simulink model "APLRL2D_avoidance_version"  (R2020a)
settings: Solver=ode23t  StartTime=0.0  StopTime=Tf  RelTol=1e-2  EnableMultiTasking=on
PreLoadFcn:
  | robotParametersRL
undefined symbols (not defined in the file or in its folder): Angular, Linear, Pose
libraries: robotlib x12, simulink x6, sharedtransform x1, rllib x1
(part 1 of 2)
settings Model: EnablePacing=on  Creator=scastro  LastModifiedBy=apl
settings SolverCC: ZeroCrossAlgorithm=Adaptive
settings DataIOCC: SaveOutput=off  SignalLogging=off  DSMLogging=off  SaveTime=off  ReturnWorkspaceOutputs=off  OutputTimes=0:0.01:10
settings OptimizationCC: LifeSpan=inf
settings DebuggingCC: MaxConsecutiveZCsMsg=warning  IgnoredZcDiagnostic=none  ParameterPrecisionLossMsg=none  AllowSymbolicDim=off  SFUnexpectedBacktrackingDiag=warning  SFNoUnconditionalDefaultTransitionDiag=warning  SFExecutionAtInitializationDiag=none  UnitsInconsistencyMsg=none  ArithmeticOperatorsInVariantConditions=warning
settings SFSimCC: SimUseLocalCustomCode=off  CustomCodeUndefinedFunction=UseInterfaceOnly
settings RTWCC: RTWUseLocalCustomCode=off
settings CodeAppCC: StateflowObjectComments=on
settings GRTTargetCC: TargetLangStandard=C89/C90 (ANSI)
settings ConfigComp: CovMetricSettings=dw  CovHtmlReporting=on  CovSaveCumulativeToWorkspaceVar=on  CovSaveSingleToWorkspaceVar=on  CovExternalEMLEnable=off  CovSFcnEnable=off
settings SimscapeCC: SimscapeNormalizeSystem=off  SimscapeLogOpenViewer=on  SimscapeLogLimitData=off  SimscapeLogDataHistory=10000
settings ConfigurationSet: Description=SimMechanics 2G
settings DiagnosticsConfigSet: SimMechanicsRigidlyBoundBlock=none
settings ExplorerConfigSet: InternalSimMechanicsExplorerSettings="<ExplorerConfiguration><canonicalview>default</canonicalview><AnimationSetting><BasePlaybackSpeed>1.0</BasePlaybackSpeed><PlaybackSpeedFactor>1.0</PlaybackSpeedFactor></AnimationSetting><TilePanel><TileInfo><Tiles Columns=\"1\" Count=\"1\" Rows=\"1\"><Column Weight=\"1\"/><Row Weight=\"1\"/><Tile Height=\"1\" Width=\"1\" X=\"0\" Y=\"0\"/></Tiles></TileInfo><SceneInfo><SceneViewer><BGColor><R>0.60000002384185791</R><G>0.60000002384185791</G><B>0.60000002384185791</B></BGColor><Camera><DoPerspective>off</DoPerspective><Position><X>8.91370771296205788</X><Y>-7.80792633437846995</Y><Z>7.38233363180041291</Z></Position><Center><X>2.84109241733315354</X><Y>0.225363634109725985</Y><Z>-0.303011043015117276</Z></Center><Up><X>-0.335329266167064488</X><Y>0.506481739462631531</Y><Z>0.79437430147428989</Z></Up><ViewLimDist>1</ViewLimDist><YLim>1.70039015453236564</YLim><XLim>2.75119305901865907</XLim></Camera></SceneViewer></SceneInfo></TilePanel><MechEditorPanel><Cameras/><GfxPanelCameraMap/><VideoCreator><PlaybackSpeedRatio>1.0</PlaybackSpeedRatio><FrameRate>30</FrameRate><VideoFormat>Motion JPEG AVI</VideoFormat><FrameSize>auto</FrameSize></VideoCreator></MechEditorPanel></ExplorerConfiguration>"

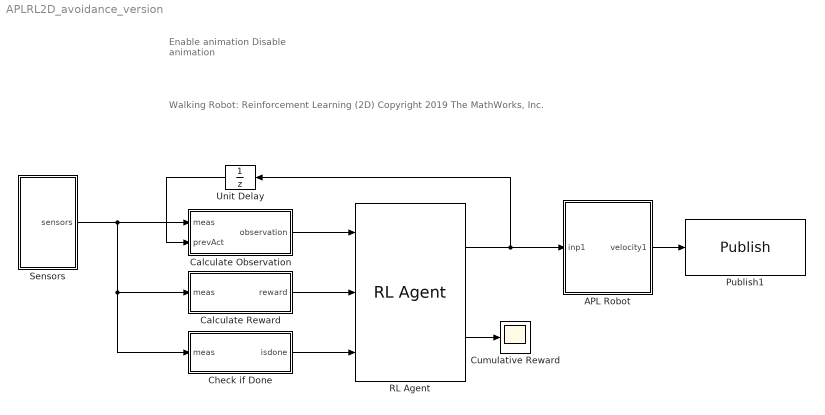
== system APLRL2D_avoidance_version ==
  note: Enable animation
      |
      | Disable animation
  note: Walking Robot: Reinforcement Learning (2D)
      |
      | Copyright 2019 The MathWorks, Inc.
  APL Robot : Subsystem
  Calculate Observation : Subsystem
  Calculate Reward : Subsystem
  Check if Done : Subsystem
  Cumulative Reward : Scope
  Publish1 : robotlib/Publish  topicSource=Select from ROS network  topic=/cmd_vel  messageType=geometry_msgs/Twist  messageQueueLength=10
  RL Agent : rllib/RL Agent  Agent=agent  ProvideReward=on  ProvideIsDone=on  ProvideCumRwd=on  TreatAsDirectFeedthrough=on  CollectLoggedSignals=on  CollectModelStates=on
      settings: SourceProductName=Reinforcement Learning
  Sensors : Subsystem
  Unit Delay : UnitDelay  SampleTime=-1  HasFrameUpgradeWarning=on
  wires:
  Calculate Reward/1(reward) -> RL Agent/2
  Calculate Observation/1(observation) -> RL Agent/1
  Check if Done/1(isdone) -> RL Agent/3
  RL Agent/2 -> Cumulative Reward/1
  Unit Delay/1 -> Calculate Observation/2(prevAct)
  APL Robot/1(velocity1) -> Publish1/1
  RL Agent/1 -> Unit Delay/1, APL Robot/1(inp1)
  Sensors/1(sensors) -> Check if Done/1(meas), Calculate Reward/1(meas), Calculate Observation/1(meas)

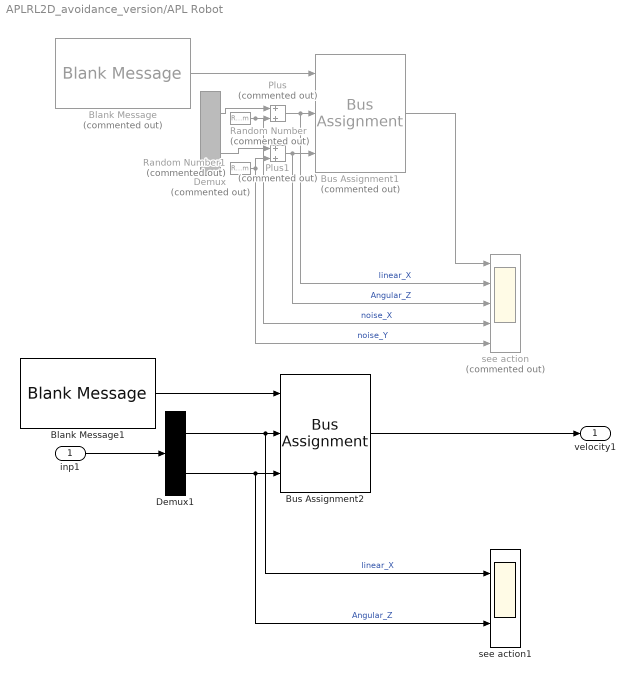
== system APLRL2D_avoidance_version/APL Robot ==
  inp1 : Inport
  Blank Message : robotlib/Blank Message  Commented=on  messageClass=Message  entityType=geometry_msgs/Twist  messageType=geometry_msgs/Twist  SampleTime=inf
  Blank Message1 : robotlib/Blank Message  messageClass=Message  entityType=geometry_msgs/Twist  messageType=geometry_msgs/Twist  SampleTime=inf
  Bus Assignment1 : BusAssignment  Commented=on  AssignedSignals=Linear.X,Angular.Z
  Bus Assignment2 : BusAssignment  AssignedSignals=Linear.X,Angular.Z
  Demux : Demux  Commented=on  Outputs=2
  Demux1 : Demux  Outputs=2
  Plus : Sum  Commented=on
  Plus1 : Sum  Commented=on
  Random Number : RandomNumber  Commented=on  Variance=0.005625  Seed=1  SampleTime=0.1
  Random Number1 : RandomNumber  Commented=on  Variance=0.005625  SampleTime=0.1
  see action : Scope  Commented=on  NumInputPorts=5
  see action1 : Scope  NumInputPorts=2
  velocity1 : Outport  VectorParamsAs1DForOutWhenUnconnected=off
  wires:
  Demux/2 -> Plus1/1
  Demux/1 -> Plus/1
  Blank Message/1 -> Bus Assignment1/1
  Bus Assignment1/1 -> see action/1
  Plus/1 -> see action/2, Bus Assignment1/2  "linear_X"
  Random Number/1 -> see action/4, Plus/2  "noise_X"
  Random Number1/1 -> see action/5, Plus1/2  "noise_Y"
  Plus1/1 -> see action/3, Bus Assignment1/3  "Angular_Z"
  Demux1/1 -> see action1/1, Bus Assignment2/2  "linear_X"
  Demux1/2 -> see action1/2, Bus Assignment2/3  "Angular_Z"
  Blank Message1/1 -> Bus Assignment2/1
  Bus Assignment2/1 -> velocity1/1
  inp1/1 -> Demux1/1

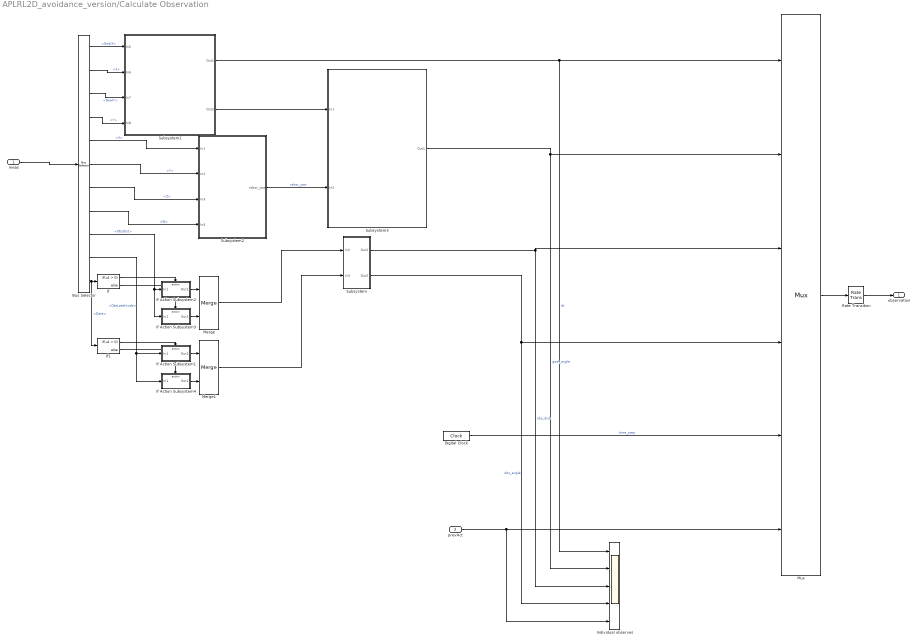
== system APLRL2D_avoidance_version/Calculate Observation ==
  meas : Inport
  prevAct : Inport  Port=2
  Bus Selector : BusSelector  OutputSignals=signal2.GoalX,signal3.Pose.Pose.Position.X,signal2.GoalY,signal3.Pose.Pose.Position.Y,signal3.Pose.Pose.Orientation.X,signal3.Pose.Pose.Orientation.Y,signal3.Pose.Pose.Orientation.Z,signal3.Pose.Pose.Orientation.W,signal2.ObsDist,signal2.ObsLatelitude,signal1.Data
  Digital Clock : DigitalClock  SampleTime=0.1
  If : If
  If Action Subsystem1 : Subsystem  TreatAsAtomicUnit=on
  If Action Subsystem2 : Subsystem  TreatAsAtomicUnit=on
  If Action Subsystem3 : Subsystem  TreatAsAtomicUnit=on
  If Action Subsystem4 : Subsystem  TreatAsAtomicUnit=on
  If1 : If
  Individual observes : Scope  NumInputPorts=5
  Merge : Merge
  Merge1 : Merge
  Mux : Mux  Inputs=6
  Rate Transition : RateTransition
  Subsystem : Subsystem
  Subsystem1 : Subsystem
  Subsystem2 : Subsystem
  Subsystem3 : Subsystem
  observation : Outport  VectorParamsAs1DForOutWhenUnconnected=off
  wires:
  meas/1 -> Bus Selector/1
  Mux/1 -> Rate Transition/1
  prevAct/1 -> Individual observes/5, Mux/6
  Rate Transition/1 -> observation/1
  Digital Clock/1 -> Mux/5  "time_step"
  Bus Selector/2 -> Subsystem1/2(In6)  "<X>"
  Bus Selector/4 -> Subsystem1/4(In8)  "<Y>"
  Bus Selector/1 -> Subsystem1/1(In5)  "<GoalX>"
  Bus Selector/3 -> Subsystem1/3(In7)  "<GoalY>"
  Subsystem1/1(Out1) -> Individual observes/1, Mux/1  "dt"
  Bus Selector/8 -> Subsystem2/4(In4)  "<W>"
  Bus Selector/7 -> Subsystem2/3(In3)  "<Z>"
  Bus Selector/6 -> Subsystem2/2(In2)  "<Y>"
  Bus Selector/5 -> Subsystem2/1(In1)  "<X>"
  Subsystem1/2(Out2) -> Subsystem3/1(In1)
  Subsystem3/1(Out1) -> Individual observes/2, Mux/2  "goal_angle"
  Bus Selector/9 -> If Action Subsystem3/1(In1), If Action Subsystem2/1(In1)  "<ObsDist>"
  Subsystem/1(Out1) -> Individual observes/3, Mux/3  "obs_dist"
  Subsystem/2(Out2) -> Individual observes/4, Mux/4  "obs_angle"
  Subsystem2/1(robot_yaw) -> Subsystem3/2(In2)  "robot_yaw"
  Merge/1 -> Subsystem/1(In2)
  Merge1/1 -> Subsystem/2(In3)
  Bus Selector/11 -> If1/1, If/1  "<Data>"
  If/1 -> If Action Subsystem2/Action
  If/2 -> If Action Subsystem3/Action
  If Action Subsystem2/1(Out1) -> Merge/1
  If Action Subsystem3/1(Out1) -> Merge/2
  If Action Subsystem1/1(Out1) -> Merge1/1
  If1/2 -> If Action Subsystem4/Action
  If Action Subsystem4/1(Out1) -> Merge1/2
  If1/1 -> If Action Subsystem1/Action
  Bus Selector/10 -> If Action Subsystem1/1(In1), If Action Subsystem4/1(In1)  "<ObsLatelitude>"

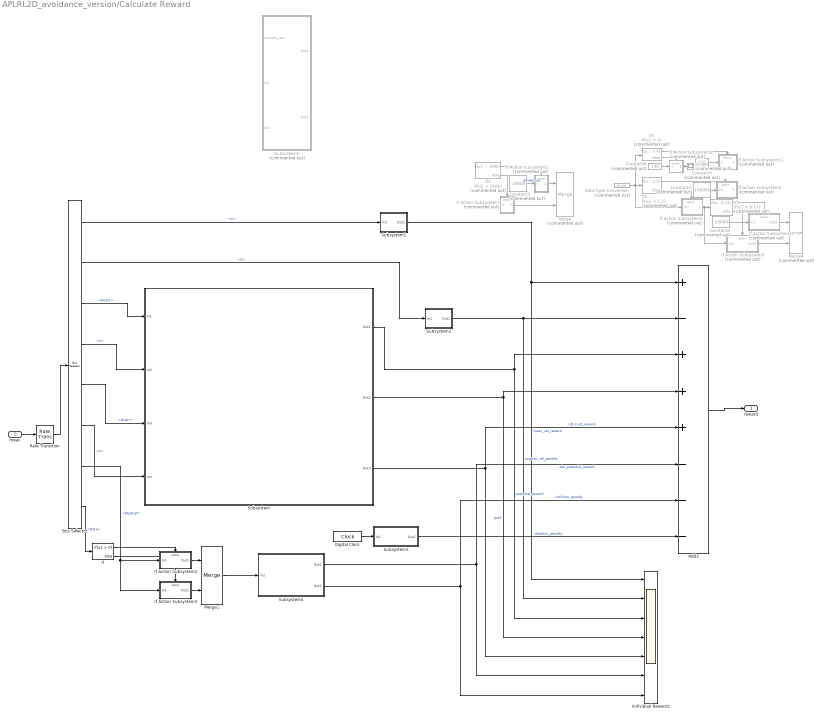
== system APLRL2D_avoidance_version/Calculate Reward ==
  meas : Inport
  Add2 : Sum  Inputs=+-+++---
  Bus Selector : BusSelector  OutputSignals=signal3.Twist.Twist.Linear.X,signal3.Twist.Twist.Angular.Z,signal2.GoalX,signal3.Pose.Pose.Position.X,signal2.GoalY,signal3.Pose.Pose.Position.Y,signal2.ObsDist,signal1.Data
  Constant2 : Constant  Commented=on  Value=100000
  Constant3 : Constant  Commented=on  Value=-10000
  Constant4 : Constant  Commented=on  Value=10000
  Constant5 : Constant  Commented=on  Value=100
  Constant6 : Constant  Commented=on  Value=100
  Data Type Conversion : DataTypeConversion  Commented=on  OutDataTypeStr=double
  Digital Clock : DigitalClock  SampleTime=0.1
  If : If
  If Action Subsystem1 : Subsystem  Commented=on  TreatAsAtomicUnit=on
  If Action Subsystem10 : Subsystem  Commented=on  TreatAsAtomicUnit=on
  If Action Subsystem11 : Subsystem  Commented=on  TreatAsAtomicUnit=on
  If Action Subsystem2 : Subsystem  TreatAsAtomicUnit=on
  If Action Subsystem3 : Subsystem  TreatAsAtomicUnit=on
  If Action Subsystem5 : Subsystem  Commented=on  TreatAsAtomicUnit=on
  If Action Subsystem6 : Subsystem  Commented=on  TreatAsAtomicUnit=on
  If Action Subsystem7 : Subsystem  Commented=on  TreatAsAtomicUnit=on
  If Action Subsystem8 : Subsystem  Commented=on  TreatAsAtomicUnit=on
  If Action Subsystem9 : Subsystem  Commented=on  TreatAsAtomicUnit=on
  If2 : If  Commented=on  IfExpression=u1 < 1.2
  If3 : If  Commented=on  IfExpression=u1 < 1000
  If4 : If  Commented=on  IfExpression=u1 > 8.15
  If5 : If  Commented=on  IfExpression=u1 < 4
  Individual Rewards : Scope  NumInputPorts=7
  Merge : Merge  Commented=on
  Merge1 : Merge
  Merge4 : Merge  Commented=on
  Rate Transition : RateTransition  OutPortSampleTime=Ts
  Scope : Scope  Commented=on
  Subsystem : Subsystem
  Subsystem1 : Subsystem
  Subsystem2 : Subsystem
  Subsystem3 : Subsystem
  Subsystem4 : Subsystem
  Subsystem5 : Subsystem  Commented=on
  reward : Outport  VectorParamsAs1DForOutWhenUnconnected=off
  wires:
  meas/1 -> Rate Transition/1
  Rate Transition/1 -> Bus Selector/1
  Add2/1 -> reward/1
  Subsystem1/1(Out1) -> Individual Rewards/1, Add2/1  "linear_vel_reward"
  If2/2 -> If Action Subsystem5/Action
  If2/1 -> If Action Subsystem6/Action
  Constant2/1 -> If Action Subsystem6/1(In1)
  If3/1 -> If Action Subsystem1/Action
  If3/2 -> If Action Subsystem7/Action
  Constant3/1 -> If Action Subsystem1/1(In1)  "dangerous"
  If Action Subsystem1/1(Out1) -> Merge/1
  If Action Subsystem7/1(Out1) -> Merge/2
  If Action Subsystem5/1(Out1) -> If Action Subsystem9/1(In1), If4/1
  If4/1 -> If Action Subsystem10/Action
  Constant4/1 -> If Action Subsystem10/1(In1)
  If4/2 -> If Action Subsystem9/Action
  If Action Subsystem10/1(Out1) -> Merge4/1
  If Action Subsystem9/1(Out1) -> Merge4/2
  Data Type Conversion/1 -> If5/1, If2/1, If Action Subsystem5/1(In1)
  If5/2 -> If Action Subsystem8/Action
  If5/1 -> If Action Subsystem11/Action
  Constant5/1 -> If Action Subsystem11/1(In1)
  Constant6/1 -> If Action Subsystem8/1(In1)
  If Action Subsystem8/1(Out1) -> Scope/1
  Subsystem/1(Out1) -> Individual Rewards/3, Add2/3  "potential_reward"
  Subsystem/2(Out2) -> Individual Rewards/4, Add2/4  "goal!"
  Bus Selector/3 -> Subsystem/1(In1)  "<GoalX>"
  Bus Selector/5 -> Subsystem/3(In3)  "<GoalY>"
  Bus Selector/4 -> Subsystem/2(In2)  "<X>"
  Subsystem3/1(Out1) -> Add2/8  "duration_penalty"
  Subsystem/3(Out3) -> Individual Rewards/5, Add2/5  "(dt-1)-dt_reward"
  Subsystem2/1(Out1) -> Individual Rewards/2, Add2/2  "angular_vel_penalty"
  Digital Clock/1 -> Subsystem3/1(In1)
  Bus Selector/7 -> If Action Subsystem2/1(In1), If Action Subsystem3/1(In1)  "<ObsDist>"
  Subsystem4/1(Out1) -> Add2/6, Individual Rewards/6  "obs_potential_reward"
  Subsystem4/2(Out2) -> Add2/7, Individual Rewards/7  "collision_penalty"
  Merge1/1 -> Subsystem4/1(In2)
  Bus Selector/6 -> Subsystem/4(In4)  "<Y>"
  Bus Selector/1 -> Subsystem1/1(In1)  "<X>"
  Bus Selector/2 -> Subsystem2/1(In1)  "<Z>"
  If Action Subsystem2/1(Out1) -> Merge1/1
  If/2 -> If Action Subsystem3/Action
  If Action Subsystem3/1(Out1) -> Merge1/2
  If/1 -> If Action Subsystem2/Action
  Bus Selector/8 -> If/1  "<Data>"

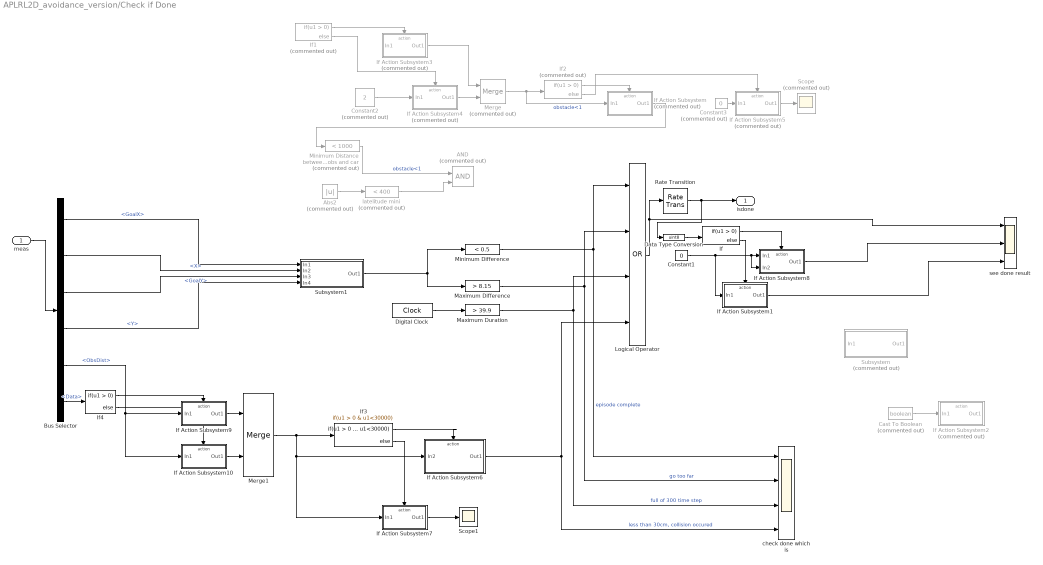
== system APLRL2D_avoidance_version/Check if Done ==
  meas : Inport
  AND : Logic  Commented=on  IconShape=distinctive  AllPortsSameDT=off  OutDataTypeStr=boolean
  Abs2 : Abs  Commented=on
  Bus Selector : BusSelector  OutputSignals=signal2.GoalX,signal3.Pose.Pose.Position.X,signal2.GoalY,signal3.Pose.Pose.Position.Y,signal2.ObsDist,signal1.Data
  Cast To Boolean : DataTypeConversion  Commented=on  OutDataTypeStr=boolean
  Constant1 : Constant  Value=0
  Constant2 : Constant  Commented=on  Value=2
  Constant3 : Constant  Commented=on  Value=0
  Data Type Conversion : DataTypeConversion  OutDataTypeStr=uint8
  Digital Clock : DigitalClock  SampleTime=0.1
  If : If
  If Action Subsystem : Subsystem  Commented=on  TreatAsAtomicUnit=on
  If Action Subsystem1 : Subsystem  TreatAsAtomicUnit=on
  If Action Subsystem10 : Subsystem  TreatAsAtomicUnit=on
  If Action Subsystem2 : Subsystem  Commented=on  TreatAsAtomicUnit=on
  If Action Subsystem3 : Subsystem  Commented=on  TreatAsAtomicUnit=on
  If Action Subsystem4 : Subsystem  Commented=on  TreatAsAtomicUnit=on
  If Action Subsystem5 : Subsystem  Commented=on  TreatAsAtomicUnit=on
  If Action Subsystem6 : Subsystem  TreatAsAtomicUnit=on
  If Action Subsystem7 : Subsystem  TreatAsAtomicUnit=on
  If Action Subsystem8 : Subsystem  TreatAsAtomicUnit=on
  If Action Subsystem9 : Subsystem  TreatAsAtomicUnit=on
  If1 : If  Commented=on
  If2 : If  Commented=on
  If3 : If  IfExpression=u1 > 0 & u1<30000
  If4 : If
  Logical Operator : Logic  Operator=OR  Inputs=4  AllPortsSameDT=off  OutDataTypeStr=boolean
  Maximum Difference : simulink/Logic and Bit Operations/Compare To Constant  relop=>  const=8.15  OutDataTypeStr=boolean
  Maximum Duration : simulink/Logic and Bit Operations/Compare To Constant  relop=>  const=39.9  OutDataTypeStr=boolean
  Merge : Merge  Commented=on
  Merge1 : Merge
  Minimum Difference : simulink/Logic and Bit Operations/Compare To Constant  relop=<  const=0.5  OutDataTypeStr=boolean
  Minimum Distance between obs and car : simulink/Logic and Bit Operations/Compare To Constant  Commented=on  relop=<  const=1000  OutDataTypeStr=boolean
  Rate Transition : RateTransition
  Scope : Scope  Commented=on
  Scope1 : Scope
  Subsystem : Subsystem  Commented=on
  Subsystem1 : Subsystem
  check done which is : Scope  NumInputPorts=4
  latelitude mini : simulink/Logic and Bit Operations/Compare To Constant  Commented=on  relop=<  const=400  OutDataTypeStr=boolean
  see done result : Scope  NumInputPorts=3
  isdone : Outport  VectorParamsAs1DForOutWhenUnconnected=off
  wires:
  Logical Operator/1 -> Rate Transition/1, see done result/1
  meas/1 -> Bus Selector/1
  Rate Transition/1 -> Data Type Conversion/1, isdone/1
  Data Type Conversion/1 -> If/1
  Subsystem1/1(Out1) -> Minimum Difference/1, Maximum Difference/1
  Minimum Difference/1 -> check done which is/1, Logical Operator/1  "episode complete"
  Cast To Boolean/1 -> If Action Subsystem2/1(In1)
  Maximum Difference/1 -> check done which is/2, Logical Operator/2  "go too far"
  Digital Clock/1 -> Maximum Duration/1
  Maximum Duration/1 -> check done which is/3, Logical Operator/3  "full of 300 time step"
  If1/1 -> If Action Subsystem3/Action
  If1/2 -> If Action Subsystem4/Action
  Constant2/1 -> If Action Subsystem4/1(In1)
  If Action Subsystem4/1(Out1) -> Merge/2
  If Action Subsystem3/1(Out1) -> Merge/1
  Merge/1 -> If Action Subsystem/1(In1), If2/1  "obstacle<1"
  If2/1 -> If Action Subsystem/Action
  If2/2 -> If Action Subsystem5/Action
  If Action Subsystem/1(Out1) -> Minimum Distance between obs and car/1
  Constant3/1 -> If Action Subsystem5/1(In1)
  If Action Subsystem5/1(Out1) -> Scope/1
  latelitude mini/1 -> AND/2
  Abs2/1 -> latelitude mini/1
  Minimum Distance between obs and car/1 -> AND/1  "obstacle<1"
  Bus Selector/1 -> Subsystem1/1(In1)  "<GoalX>"
  Bus Selector/2 -> Subsystem1/2(In2)  "<X>"
  Bus Selector/3 -> Subsystem1/3(In3)  "<GoalY>"
  Bus Selector/4 -> Subsystem1/4(In4)  "<Y>"
  If Action Subsystem6/1(Out1) -> Logical Operator/4, check done which is/4  "less than 30cm, collision occured"
  If Action Subsystem7/1(Out1) -> Scope1/1
  If/1 -> If Action Subsystem8/Action
  Constant1/1 -> If Action Subsystem1/1(In1), If Action Subsystem8/2(In2), If Action Subsystem8/1(In1)
  If Action Subsystem8/1(Out1) -> see done result/2
  If Action Subsystem1/1(Out1) -> see done result/3
  If/2 -> If Action Subsystem1/Action
  Merge1/1 -> If Action Subsystem7/1(In1), If Action Subsystem6/1(In2), If3/1
  If3/1 -> If Action Subsystem6/Action
  If3/2 -> If Action Subsystem7/Action
  If4/1 -> If Action Subsystem9/Action
  If Action Subsystem9/1(Out1) -> Merge1/1
  If4/2 -> If Action Subsystem10/Action
  Bus Selector/5 -> If Action Subsystem9/1(In1), If Action Subsystem10/1(In1)  "<ObsDist>"
  If Action Subsystem10/1(Out1) -> Merge1/2
  Bus Selector/6 -> If4/1  "<Data>"

== system APLRL2D_avoidance_version/Sensors ==
  Bus Creator : BusCreator  Inputs=3
  Rate Transition : RateTransition
  Read Objects Number : Subsystem  TreatAsAtomicUnit=on
  Read Odometry1 : Subsystem  TreatAsAtomicUnit=on
  Read Preprocess data : Subsystem  TreatAsAtomicUnit=on
  Subscribe : robotlib/Subscribe  topicSource=Select from ROS network  topic=/apl_pub  messageType=relative_angle_nb/Apl_kai  sampleTime=-1  messageQueueLength=1
  Subscribe1 : robotlib/Subscribe  topicSource=Select from ROS network  topic=/rtabmap/odom  messageType=nav_msgs/Odometry  sampleTime=0.1  messageQueueLength=1
  Subscribe4 : robotlib/Subscribe  topicSource=Select from ROS network  topic=/darknet_ros/found_object  messageType=std_msgs/Int8  sampleTime=-1  messageQueueLength=1
  sensors : Outport  VectorParamsAs1DForOutWhenUnconnected=off
  wires:
  Subscribe1/1 -> Read Odometry1/Enable
  Subscribe1/2 -> Read Odometry1/1(msg)
  Bus Creator/1 -> Rate Transition/1
  Rate Transition/1 -> sensors/1
  Subscribe4/1 -> Read Objects Number/Enable
  Subscribe4/2 -> Read Objects Number/1(msg)
  Subscribe/2 -> Read Preprocess data/1(msg)
  Subscribe/1 -> Read Preprocess data/Enable
  Read Objects Number/1(obs_num) -> Bus Creator/1
  Read Odometry1/1(pose) -> Bus Creator/3
  Read Preprocess data/1(preprocess data) -> Bus Creator/2

== system APLRL2D_avoidance_version/Calculate Observation/If Action Subsystem1 ==
  In1 : Inport
  Action Port : ActionPort  ActionPortLabel=if(u1 > 0)
  Subsystem5 : Subsystem
  Out1 : Outport
  wires:
  In1/1 -> Subsystem5/1(In1)
  Subsystem5/1(Out1) -> Out1/1

== system APLRL2D_avoidance_version/Calculate Observation/If Action Subsystem2 ==
  In1 : Inport
  Action Port : ActionPort  ActionPortLabel=if(u1 > 0)
  Subsystem4 : Subsystem
  Out1 : Outport
  wires:
  In1/1 -> Subsystem4/1(In1)
  Subsystem4/1(Out1) -> Out1/1

== system APLRL2D_avoidance_version/Calculate Observation/If Action Subsystem3 ==
  In1 : Inport
  Action Port : ActionPort  ActionPortLabel=else
  Out1 : Outport
  wires:
  In1/1 -> Out1/1

== system APLRL2D_avoidance_version/Calculate Observation/If Action Subsystem4 ==
  In1 : Inport
  Action Port : ActionPort  ActionPortLabel=else
  Out1 : Outport
  wires:
  In1/1 -> Out1/1

== system APLRL2D_avoidance_version/Calculate Observation/Subsystem ==
  In2 : Inport
  In3 : Inport  Port=2
  Constant : Constant  Value=0
  Demux : Demux  Outputs=2
  If : If  IfExpression=u1 > 0 & u1<65535
  If Action Subsystem : Subsystem  TreatAsAtomicUnit=on
  If Action Subsystem1 : Subsystem  TreatAsAtomicUnit=on
  Merge : Merge
  Out1 : Outport
  Out2 : Outport  Port=2
  wires:
  Constant/1 -> If Action Subsystem1/1(In1)
  In2/1 -> If Action Subsystem/1(In2), If/1
  If/1 -> If Action Subsystem/Action
  If/2 -> If Action Subsystem1/Action
  In3/1 -> If Action Subsystem/2(In3)
  If Action Subsystem/1(Out1) -> Merge/1
  If Action Subsystem1/1(Out1) -> Merge/2
  Merge/1 -> Demux/1
  Demux/2 -> Out2/1
  Demux/1 -> Out1/1

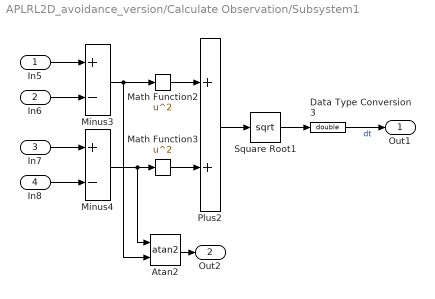
== system APLRL2D_avoidance_version/Calculate Observation/Subsystem1 ==
  In5 : Inport
  In6 : Inport  Port=2
  In7 : Inport  Port=3
  In8 : Inport  Port=4
  Atan2 : Trigonometry  Operator=atan2
  Data Type Conversion3 : DataTypeConversion  OutDataTypeStr=double
  Math Function2 : Math  Operator=square  SaturateOnIntegerOverflow=on
  Math Function3 : Math  Operator=square  SaturateOnIntegerOverflow=on
  Minus3 : Sum  Inputs=+-
  Minus4 : Sum  Inputs=+-
  Plus2 : Sum
  Square Root1 : Sqrt  SaturateOnIntegerOverflow=on
  Out1 : Outport
  Out2 : Outport  Port=2
  wires:
  Plus2/1 -> Square Root1/1
  Minus4/1 -> Atan2/1, Math Function3/1
  Minus3/1 -> Atan2/2, Math Function2/1
  Math Function3/1 -> Plus2/2
  Math Function2/1 -> Plus2/1
  In7/1 -> Minus4/1
  In5/1 -> Minus3/1
  In8/1 -> Minus4/2
  In6/1 -> Minus3/2
  Square Root1/1 -> Data Type Conversion3/1
  Data Type Conversion3/1 -> Out1/1  "dt"
  Atan2/1 -> Out2/1

== system APLRL2D_avoidance_version/Calculate Observation/Subsystem2 ==
  In1 : Inport
  In2 : Inport  Port=2
  In3 : Inport  Port=3
  In4 : Inport  Port=4
  Mux : Mux  Inputs=1
  Quaternions to Rotation Angles : sharedtransform/Quaternions to Rotation Angles  rotationOrder=ZYX  aMode=aMode
      settings: SourceProductBaseCode=AE,PW,MT,VE,VP
  Selector : Selector  InputPortWidth=3  IndexOptions=Index vector (dialog)  Indices=(3)  OutputSizes=1
  Vector Concatenate : Concatenate  NumInputs=4
  robot_yaw : Outport
  wires:
  In1/1 -> Vector Concatenate/1
  In2/1 -> Vector Concatenate/2
  In3/1 -> Vector Concatenate/3
  In4/1 -> Vector Concatenate/4
  Vector Concatenate/1 -> Quaternions to Rotation Angles/1
  Quaternions to Rotation Angles/1 -> Selector/1
  Selector/1 -> Mux/1
  Mux/1 -> robot_yaw/1

== system APLRL2D_avoidance_version/Calculate Observation/Subsystem3 ==
  In1 : Inport
  In2 : Inport  Port=2
  Constant : Constant  Value=2*pi
  If : If  IfExpression=u1 > pi  ElseIfExpressions=u1 < -pi
  If Action Subsystem : Subsystem  TreatAsAtomicUnit=on
  If Action Subsystem1 : Subsystem  TreatAsAtomicUnit=on
  If Action Subsystem2 : Subsystem  TreatAsAtomicUnit=on
  Merge : Merge  Inputs=3
  Minus : Sum  Inputs=+-
  Out1 : Outport
  wires:
  In2/1 -> Minus/2
  In1/1 -> Minus/1
  If/1 -> If Action Subsystem/Action
  If/2 -> If Action Subsystem1/Action
  If/3 -> If Action Subsystem2/Action
  Minus/1 -> If Action Subsystem2/1(In1), If Action Subsystem1/1(In1), If/1, If Action Subsystem/1(In1)
  Constant/1 -> If Action Subsystem/2(In2), If Action Subsystem1/2(In2)
  Merge/1 -> Out1/1
  If Action Subsystem2/1(Out1) -> Merge/3
  If Action Subsystem1/1(Out1) -> Merge/2
  If Action Subsystem/1(Out1) -> Merge/1

== system APLRL2D_avoidance_version/Calculate Reward/If Action Subsystem1 ==
  In1 : Inport
  Action Port : ActionPort  ActionPortLabel=if(u1 < 1000)
  Data Type Conversion : DataTypeConversion  OutDataTypeStr=double
  Out1 : Outport
  wires:
  In1/1 -> Data Type Conversion/1
  Data Type Conversion/1 -> Out1/1

== system APLRL2D_avoidance_version/Calculate Reward/If Action Subsystem10 ==
  In1 : Inport
  Action Port : ActionPort  ActionPortLabel=if(u1 > 8.15)
  Data Type Conversion : DataTypeConversion  OutDataTypeStr=double
  Out1 : Outport
  wires:
  In1/1 -> Data Type Conversion/1
  Data Type Conversion/1 -> Out1/1

== system APLRL2D_avoidance_version/Calculate Reward/If Action Subsystem11 ==
  In1 : Inport
  Action Port : ActionPort  ActionPortLabel=if(u1 < 4)
  Data Type Conversion : DataTypeConversion  OutDataTypeStr=double
  Out1 : Outport
  wires:
  In1/1 -> Data Type Conversion/1
  Data Type Conversion/1 -> Out1/1

== system APLRL2D_avoidance_version/Calculate Reward/If Action Subsystem2 ==
  In1 : Inport
  Action Port : ActionPort  ActionPortLabel=if(u1 > 0)
  Subsystem4 : Subsystem
  Out1 : Outport
  wires:
  In1/1 -> Subsystem4/1(In1)
  Subsystem4/1(Out1) -> Out1/1

== system APLRL2D_avoidance_version/Calculate Reward/If Action Subsystem3 ==
  In1 : Inport
  Action Port : ActionPort  ActionPortLabel=else
  Out1 : Outport
  wires:
  In1/1 -> Out1/1

== system APLRL2D_avoidance_version/Calculate Reward/If Action Subsystem5 ==
  In1 : Inport
  Action Port : ActionPort  ActionPortLabel=else
  Out1 : Outport
  wires:
  In1/1 -> Out1/1  "distance_reward"

== system APLRL2D_avoidance_version/Calculate Reward/If Action Subsystem6 ==
  In1 : Inport
  Action Port : ActionPort  ActionPortLabel=if(u1 < 1.2)
  Data Type Conversion : DataTypeConversion  OutDataTypeStr=double
  Out1 : Outport
  wires:
  In1/1 -> Data Type Conversion/1
  Data Type Conversion/1 -> Out1/1

== system APLRL2D_avoidance_version/Calculate Reward/If Action Subsystem7 ==
  In1 : Inport
  Action Port : ActionPort  ActionPortLabel=else
  Data Type Conversion : DataTypeConversion  OutDataTypeStr=double
  Penalty Scaling1 : Gain  Gain=0.0001
  Out1 : Outport
  wires:
  In1/1 -> Penalty Scaling1/1
  Data Type Conversion/1 -> Out1/1
  Penalty Scaling1/1 -> Data Type Conversion/1  "distance_reward"

== system APLRL2D_avoidance_version/Calculate Reward/If Action Subsystem8 ==
  In1 : Inport
  Action Port : ActionPort  ActionPortLabel=else
  Data Type Conversion : DataTypeConversion  OutDataTypeStr=double
  Out1 : Outport
  wires:
  In1/1 -> Data Type Conversion/1  "distance_reward"
  Data Type Conversion/1 -> Out1/1

== system APLRL2D_avoidance_version/Calculate Reward/If Action Subsystem9 ==
  In1 : Inport
  Action Port : ActionPort  ActionPortLabel=else
  Abs1 : Abs
  Reward Scaling : Gain  Gain=10
  Out1 : Outport
  wires:
  Abs1/1 -> Reward Scaling/1
  Reward Scaling/1 -> Out1/1  "distance_reward"
  In1/1 -> Abs1/1

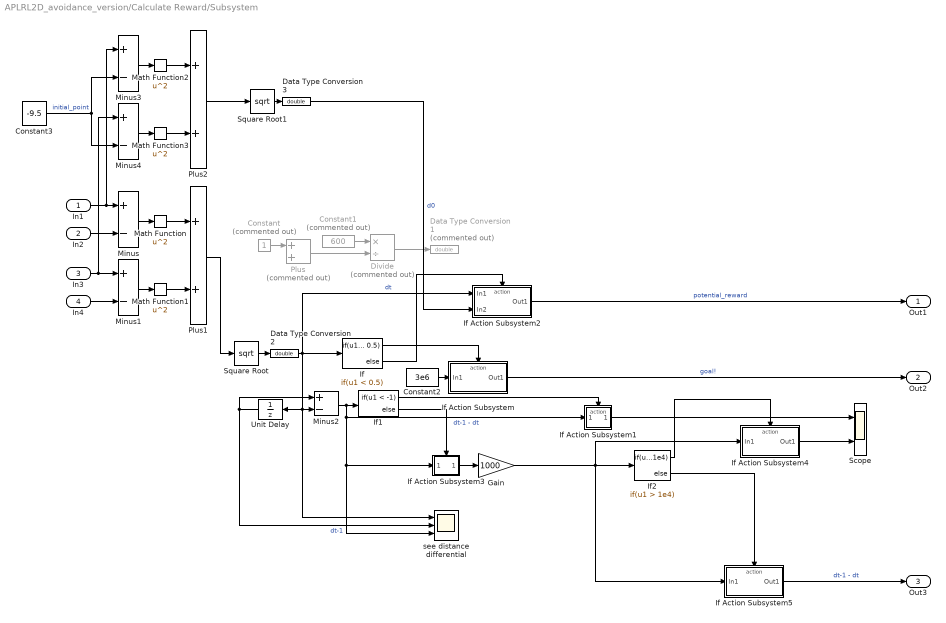
== system APLRL2D_avoidance_version/Calculate Reward/Subsystem ==
  In1 : Inport
  In2 : Inport  Port=2
  In3 : Inport  Port=3
  In4 : Inport  Port=4
  Constant : Constant  Commented=on
  Constant1 : Constant  Commented=on  Value=600
  Constant2 : Constant  Value=3e6
  Constant3 : Constant  Value=-9.5
  Data Type Conversion1 : DataTypeConversion  Commented=on  OutDataTypeStr=double
  Data Type Conversion2 : DataTypeConversion  OutDataTypeStr=double
  Data Type Conversion3 : DataTypeConversion  OutDataTypeStr=double
  Divide : Product  Commented=on  Inputs=*/
  Gain : Gain  Gain=1000
  If : If  IfExpression=u1 < 0.5
  If Action Subsystem : Subsystem  TreatAsAtomicUnit=on
  If Action Subsystem1 : Subsystem  TreatAsAtomicUnit=on
  If Action Subsystem2 : Subsystem  TreatAsAtomicUnit=on
  If Action Subsystem3 : Subsystem  TreatAsAtomicUnit=on
  If Action Subsystem4 : Subsystem  TreatAsAtomicUnit=on
  If Action Subsystem5 : Subsystem  TreatAsAtomicUnit=on
  If1 : If  IfExpression=u1 < -1
  If2 : If  IfExpression=u1 > 1e4
  Math Function{,1..3} (4 alike) : Math  Operator=square  SaturateOnIntegerOverflow=on
  Minus{,1..4} (5 alike) : Sum  Inputs=+-
  Plus : Sum  Commented=on
  Plus1 : Sum
  Plus2 : Sum
  Scope : Scope  NumInputPorts=2
  Square Root : Sqrt  SaturateOnIntegerOverflow=on
  Square Root1 : Sqrt  SaturateOnIntegerOverflow=on
  Unit Delay : UnitDelay  SampleTime=-1  HasFrameUpgradeWarning=on
  see distance differential : Scope  NumInputPorts=3
  Out1 : Outport
  Out2 : Outport  Port=2
  Out3 : Outport  Port=3
  wires:
  Plus/1 -> Divide/2
  Constant/1 -> Plus/1
  Constant1/1 -> Divide/1
  In1/1 -> Minus3/1, Minus/1
  In2/1 -> Minus/2
  In3/1 -> Minus4/1, Minus1/1
  In4/1 -> Minus1/2
  Minus1/1 -> Math Function1/1
  Minus/1 -> Math Function/1
  Math Function1/1 -> Plus1/2
  Math Function/1 -> Plus1/1
  Plus1/1 -> Square Root/1
  Divide/1 -> Data Type Conversion1/1
  Square Root/1 -> Data Type Conversion2/1
  If Action Subsystem2/1(Out1) -> Out1/1  "potential_reward"
  If/2 -> If Action Subsystem2/Action
  If Action Subsystem/1(Out1) -> Out2/1  "goal!"
  Constant2/1 -> If Action Subsystem/1(In1)
  Data Type Conversion2/1 -> If Action Subsystem2/1(In1), If/1, see distance differential/1, Unit Delay/1, Minus2/2  "dt"
  Unit Delay/1 -> see distance differential/2, Minus2/1  "dt-1"
  Minus2/1 -> see distance differential/3, If Action Subsystem3/1(In1), If Action Subsystem1/1(In1), If1/1  "dt-1 - dt"
  Gain/1 -> If Action Subsystem5/1(In1), If Action Subsystem4/1(In1), If2/1
  If1/1 -> If Action Subsystem1/Action
  If Action Subsystem1/1(Out1) -> Scope/1
  If1/2 -> If Action Subsystem3/Action
  If Action Subsystem3/1(Out1) -> Gain/1
  If/1 -> If Action Subsystem/Action
  Math Function3/1 -> Plus2/2
  Math Function2/1 -> Plus2/1
  Minus3/1 -> Math Function2/1
  Plus2/1 -> Square Root1/1
  Minus4/1 -> Math Function3/1
  Constant3/1 -> Minus3/2, Minus4/2  "initial_point"
  Square Root1/1 -> Data Type Conversion3/1
  Data Type Conversion3/1 -> If Action Subsystem2/2(In2)  "d0"
  If2/1 -> If Action Subsystem4/Action
  If Action Subsystem4/1(Out1) -> Scope/2
  If2/2 -> If Action Subsystem5/Action
  If Action Subsystem5/1(Out1) -> Out3/1  "dt-1 - dt"

== system APLRL2D_avoidance_version/Calculate Reward/Subsystem1 ==
  In1 : Inport
  Data Type Conversion1 : DataTypeConversion  OutDataTypeStr=double
  Forward Reward Scaling : Gain  Gain=66666
  Out1 : Outport
  wires:
  In1/1 -> Data Type Conversion1/1
  Data Type Conversion1/1 -> Forward Reward Scaling/1
  Forward Reward Scaling/1 -> Out1/1

== system APLRL2D_avoidance_version/Calculate Reward/Subsystem2 ==
  In1 : Inport
  Abs : Abs
  Data Type Conversion1 : DataTypeConversion  OutDataTypeStr=double
  Forward Reward Scaling : Gain  Gain=100000
  Out1 : Outport
  wires:
  In1/1 -> Data Type Conversion1/1
  Data Type Conversion1/1 -> Abs/1
  Forward Reward Scaling/1 -> Out1/1
  Abs/1 -> Forward Reward Scaling/1

== system APLRL2D_avoidance_version/Calculate Reward/Subsystem3 ==
  In1 : Inport
  Constant : Constant
  Data Type Conversion1 : DataTypeConversion  OutDataTypeStr=double
  Gain : Gain  Gain=6
  Gain1 : Gain  Gain=0.3
  Math Function : Math  SaturateOnIntegerOverflow=on
  Math Function1 : Math  SaturateOnIntegerOverflow=on
  Minus : Sum  Inputs=+-
  Out1 : Outport
  wires:
  Gain/1 -> Data Type Conversion1/1
  Math Function1/1 -> Gain/1
  Constant/1 -> Math Function/1
  Math Function/1 -> Minus/2
  Minus/1 -> Math Function1/1
  Gain1/1 -> Minus/1
  In1/1 -> Gain1/1
  Data Type Conversion1/1 -> Out1/1  "duration_penalty"

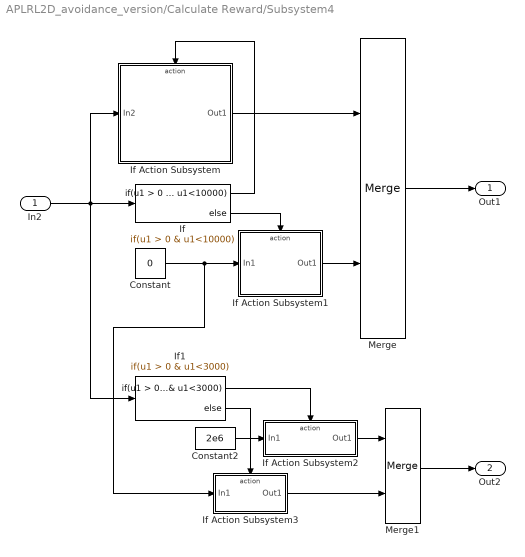
== system APLRL2D_avoidance_version/Calculate Reward/Subsystem4 ==
  In2 : Inport
  Constant : Constant  Value=0
  Constant2 : Constant  Value=2e6
  If : If  IfExpression=u1 > 0 & u1<10000
  If Action Subsystem : Subsystem  TreatAsAtomicUnit=on
  If Action Subsystem1 : Subsystem  TreatAsAtomicUnit=on
  If Action Subsystem2 : Subsystem  TreatAsAtomicUnit=on
  If Action Subsystem3 : Subsystem  TreatAsAtomicUnit=on
  If1 : If  IfExpression=u1 > 0 & u1<3000
  Merge : Merge
  Merge1 : Merge
  Out1 : Outport
  Out2 : Outport  Port=2
  wires:
  Constant/1 -> If Action Subsystem3/1(In1), If Action Subsystem1/1(In1)
  In2/1 -> If1/1, If/1, If Action Subsystem/1(In2)
  If Action Subsystem/1(Out1) -> Merge/1
  If Action Subsystem1/1(Out1) -> Merge/2
  Merge/1 -> Out1/1
  Constant2/1 -> If Action Subsystem2/1(In1)
  If Action Subsystem2/1(Out1) -> Merge1/1
  If Action Subsystem3/1(Out1) -> Merge1/2
  Merge1/1 -> Out2/1
  If/1 -> If Action Subsystem/Action
  If/2 -> If Action Subsystem1/Action
  If1/1 -> If Action Subsystem2/Action
  If1/2 -> If Action Subsystem3/Action

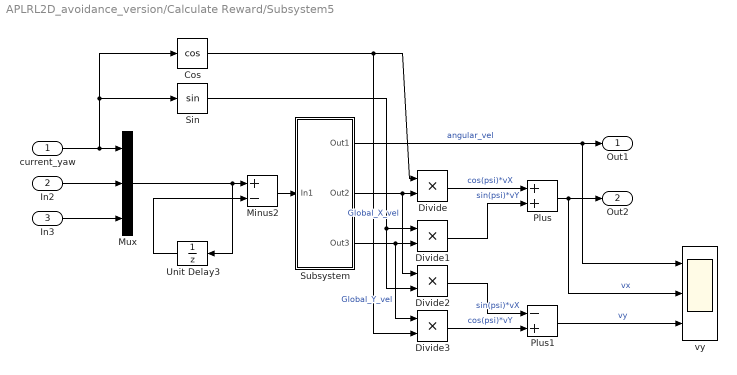
== system APLRL2D_avoidance_version/Calculate Reward/Subsystem5 ==
  current_yaw : Inport
  In2 : Inport  Port=2
  In3 : Inport  Port=3
  Cos : Trigonometry  Operator=cos
  Divide{,1..3} (4 alike) : Product  Inputs=**
  Minus2 : Sum  Inputs=+-
  Mux : Mux  Inputs=3
  Plus : Sum
  Plus1 : Sum  Inputs=-+
  Sin : Trigonometry
  Subsystem : Subsystem
  Unit Delay3 : UnitDelay  SampleTime=-1  HasFrameUpgradeWarning=on
  vy : Scope  NumInputPorts=3
  Out1 : Outport
  Out2 : Outport  Port=2
  wires:
  Unit Delay3/1 -> Minus2/2
  In3/1 -> Mux/3
  In2/1 -> Mux/2
  current_yaw/1 -> Cos/1, Sin/1, Mux/1
  Mux/1 -> Unit Delay3/1, Minus2/1
  Minus2/1 -> Subsystem/1(In1)
  Subsystem/2(Out2) -> Divide2/1, Divide/2  "Global_X_vel"
  Subsystem/3(Out3) -> Divide3/1, Divide1/2  "Global_Y_vel"
  Cos/1 -> Divide3/2, Divide/1
  Sin/1 -> Divide1/1, Divide2/2
  Divide/1 -> Plus/1  "cos(psi)*vX"
  Divide1/1 -> Plus/2  "sin(psi)*vY"
  Divide3/1 -> Plus1/2  "cos(psi)*vY"
  Divide2/1 -> Plus1/1  "sin(psi)*vX"
  Plus1/1 -> vy/3  "vy"
  Plus/1 -> vy/2, Out2/1  "vx"
  Subsystem/1(Out1) -> vy/1, Out1/1  "angular_vel"

== system APLRL2D_avoidance_version/Check if Done/If Action Subsystem ==
  In1 : Inport
  Action Port : ActionPort  ActionPortLabel=if(u1 > 0)
  Out1 : Outport
  wires:
  In1/1 -> Out1/1

== system APLRL2D_avoidance_version/Check if Done/If Action Subsystem1 ==
  In1 : Inport
  Action Port : ActionPort  ActionPortLabel=else
  Out1 : Outport
  wires:
  In1/1 -> Out1/1

== system APLRL2D_avoidance_version/Check if Done/If Action Subsystem10 ==
  In1 : Inport
  Action Port : ActionPort  ActionPortLabel=else
  Out1 : Outport
  wires:
  In1/1 -> Out1/1

== system APLRL2D_avoidance_version/Check if Done/If Action Subsystem2 ==
  In1 : Inport
  Action Port : ActionPort  ActionPortLabel=if(u1 > 0)
  Blank Message : robotlib/Blank Message  messageClass=Service Request  entityType=std_srvs/Empty  messageType=std_srvs/EmptyRequest  SampleTime=inf
  Bus Assignment : BusAssignment  AssignedSignals=SL_DummyData
  Bus Selector1 : BusSelector  OutputSignals=SL_DummyData
  Call Service : robotlib/Call Service  topicSource=Specify your own  service=/gazebo/reset_simulation  serviceType=std_srvs/Empty  connectionTimeout=5  keepPersistent=on  ShowErrorCodeOutput=off
      settings: SourceProductBaseCode=RR
  Scope : Scope
  Out1 : Outport
  wires:
  In1/1 -> Out1/1, Bus Assignment/2
  Bus Selector1/1 -> Scope/1  "<SL_DummyData>"
  Blank Message/1 -> Bus Assignment/1
  Bus Assignment/1 -> Call Service/1
  Call Service/1 -> Bus Selector1/1

== system APLRL2D_avoidance_version/Check if Done/If Action Subsystem3 ==
  In1 : Inport
  Action Port : ActionPort  ActionPortLabel=if(u1 > 0)
  Abs3 : Abs
  Data Type Conversion : DataTypeConversion  OutDataTypeStr=double
  Out1 : Outport
  wires:
  In1/1 -> Data Type Conversion/1
  Data Type Conversion/1 -> Abs3/1
  Abs3/1 -> Out1/1

== system APLRL2D_avoidance_version/Check if Done/If Action Subsystem4 ==
  In1 : Inport
  Action Port : ActionPort  ActionPortLabel=else
  Penalty Scaling1 : Gain  Gain=10000
  Out1 : Outport
  wires:
  In1/1 -> Penalty Scaling1/1
  Penalty Scaling1/1 -> Out1/1  "distance_reward"

== system APLRL2D_avoidance_version/Check if Done/If Action Subsystem5 ==
  In1 : Inport
  Action Port : ActionPort  ActionPortLabel=else
  Out1 : Outport
  wires:
  In1/1 -> Out1/1

== system APLRL2D_avoidance_version/Check if Done/If Action Subsystem6 ==
  In2 : Inport
  Action Port : ActionPort  ActionPortLabel=if(u1 > 0 & u1<30000)
  Gain : Gain  Gain=0.01
  obsDist_threshold : simulink/Logic and Bit Operations/Compare To Constant  relop=<  const=15  OutDataTypeStr=boolean
  Out1 : Outport
  wires:
  In2/1 -> Gain/1
  obsDist_threshold/1 -> Out1/1
  Gain/1 -> obsDist_threshold/1

== system APLRL2D_avoidance_version/Check if Done/If Action Subsystem7 ==
  In1 : Inport
  Action Port : ActionPort  ActionPortLabel=else
  Out1 : Outport
  wires:
  In1/1 -> Out1/1

== system APLRL2D_avoidance_version/Check if Done/If Action Subsystem8 ==
  In1 : Inport
  In2 : Inport  Port=2
  Action Port : ActionPort  ActionPortLabel=if(u1 > 0)
  Blank Message1 : robotlib/Blank Message  messageClass=Message  entityType=geometry_msgs/Twist  messageType=geometry_msgs/Twist  SampleTime=inf
  Bus Assignment2 : BusAssignment  AssignedSignals=Linear.X,Angular.Z
  Data Type Conversion1 : DataTypeConversion  OutDataTypeStr=double
  Data Type Conversion3 : DataTypeConversion  OutDataTypeStr=double
  Out1 : Outport
  wires:
  Blank Message1/1 -> Bus Assignment2/1
  Bus Assignment2/1 -> Out1/1
  In1/1 -> Data Type Conversion3/1
  In2/1 -> Data Type Conversion1/1
  Data Type Conversion3/1 -> Bus Assignment2/2
  Data Type Conversion1/1 -> Bus Assignment2/3

== system APLRL2D_avoidance_version/Check if Done/If Action Subsystem9 ==
  In1 : Inport
  Action Port : ActionPort  ActionPortLabel=if(u1 > 0)
  Subsystem4 : Subsystem
  Out1 : Outport
  wires:
  In1/1 -> Subsystem4/1(In1)
  Subsystem4/1(Out1) -> Out1/1

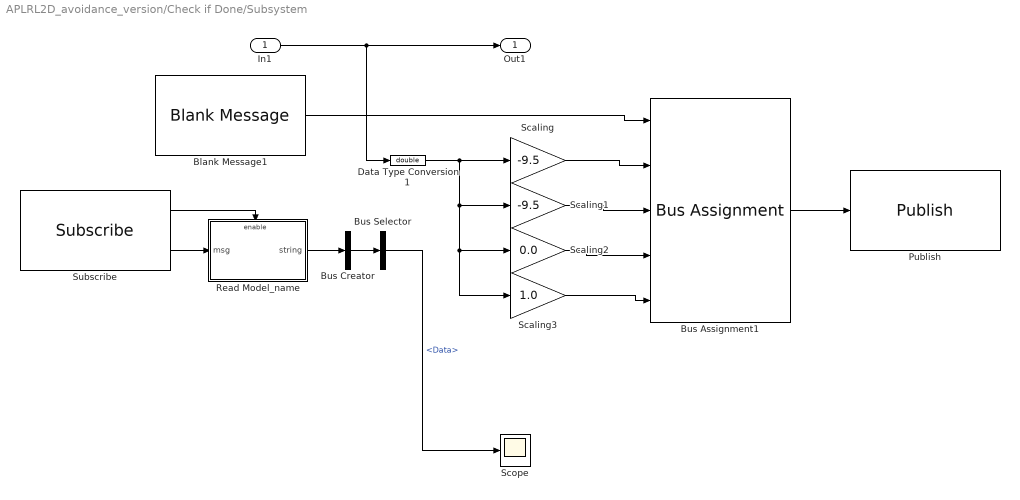
== system APLRL2D_avoidance_version/Check if Done/Subsystem ==
  In1 : Inport
  Blank Message1 : robotlib/Blank Message  messageClass=Message  entityType=gazebo_msgs/ModelState  messageType=gazebo_msgs/ModelState  SampleTime=inf
  Bus Assignment1 : BusAssignment  AssignedSignals=Pose.Position.X,Pose.Position.Y,Pose.Orientation.Z,Pose.Orientation.W
  Bus Creator : BusCreator  Inputs=1
  Bus Selector : BusSelector  OutputSignals=signal1.Data
  Data Type Conversion1 : DataTypeConversion  OutDataTypeStr=double
  Publish : robotlib/Publish  topicSource=Specify your own  topic=/gazebo/set_model_state  messageType=gazebo_msgs/ModelState  messageQueueLength=1
  Read Model_name : Subsystem  TreatAsAtomicUnit=on
  Scaling : Gain  Gain=-9.5
  Scaling1 : Gain  Gain=-9.5
  Scaling2 : Gain  Gain=0.0
  Scaling3 : Gain  Gain=1.0
  Scope : Scope
  Subscribe : robotlib/Subscribe  topicSource=Select from ROS network  topic=/string_for_simulink  messageType=std_msgs/String  sampleTime=-1  messageQueueLength=1
  Out1 : Outport
  wires:
  Bus Assignment1/1 -> Publish/1
  Data Type Conversion1/1 -> Scaling/1, Scaling3/1, Scaling2/1, Scaling1/1
  Blank Message1/1 -> Bus Assignment1/1
  Scaling1/1 -> Bus Assignment1/3
  Scaling2/1 -> Bus Assignment1/4
  Scaling3/1 -> Bus Assignment1/5
  In1/1 -> Data Type Conversion1/1, Out1/1
  Scaling/1 -> Bus Assignment1/2
  Read Model_name/1(string) -> Bus Creator/1
  Subscribe/1 -> Read Model_name/Enable
  Subscribe/2 -> Read Model_name/1(msg)
  Bus Creator/1 -> Bus Selector/1
  Bus Selector/1 -> Scope/1  "<Data>"

== system APLRL2D_avoidance_version/Check if Done/Subsystem1 ==
  In1 : Inport
  In2 : Inport  Port=2
  In3 : Inport  Port=3
  In4 : Inport  Port=4
  Math Function : Math  Operator=square  SaturateOnIntegerOverflow=on
  Math Function1 : Math  Operator=square  SaturateOnIntegerOverflow=on
  Minus : Sum  Inputs=+-
  Minus1 : Sum  Inputs=+-
  Plus1 : Sum
  Square Root : Sqrt  SaturateOnIntegerOverflow=on
  Out1 : Outport
  wires:
  In1/1 -> Minus/1
  In2/1 -> Minus/2
  In3/1 -> Minus1/1
  In4/1 -> Minus1/2
  Minus1/1 -> Math Function1/1
  Minus/1 -> Math Function/1
  Math Function1/1 -> Plus1/2
  Math Function/1 -> Plus1/1
  Plus1/1 -> Square Root/1
  Square Root/1 -> Out1/1

== system APLRL2D_avoidance_version/Sensors/Read Objects Number ==
  msg : Inport
  Enable : EnablePort
  obs_num : Outport
  wires:
  msg/1 -> obs_num/1

== system APLRL2D_avoidance_version/Sensors/Read Odometry1 ==
  msg : Inport
  Enable : EnablePort
  pose : Outport
  wires:
  msg/1 -> pose/1

== system APLRL2D_avoidance_version/Sensors/Read Preprocess data ==
  msg : Inport
  Enable : EnablePort
  preprocess data : Outport
  wires:
  msg/1 -> preprocess data/1

== system APLRL2D_avoidance_version/Calculate Observation/If Action Subsystem1/Subsystem5 ==
  In1 : Inport
  If : If
  If Action Subsystem : Subsystem  TreatAsAtomicUnit=on
  If Action Subsystem1 : Subsystem  TreatAsAtomicUnit=on
  Merge : Merge
  Unit Delay : UnitDelay  SampleTime=-1  HasFrameUpgradeWarning=on
  Out1 : Outport
  wires:
  In1/1 -> Unit Delay/1, If Action Subsystem/1(In1), If/1
  If/1 -> If Action Subsystem/Action
  If/2 -> If Action Subsystem1/Action
  Unit Delay/1 -> If Action Subsystem1/1(In1)
  If Action Subsystem1/1(Out1) -> Merge/2
  If Action Subsystem/1(Out1) -> Merge/1
  Merge/1 -> Out1/1

== system APLRL2D_avoidance_version/Calculate Observation/If Action Subsystem2/Subsystem4 ==
  In1 : Inport
  Data Type Conversion2 : DataTypeConversion  OutDataTypeStr=uint16
  Gain : Gain  Gain=10
  If : If
  If Action Subsystem : Subsystem  TreatAsAtomicUnit=on
  If Action Subsystem1 : Subsystem  TreatAsAtomicUnit=on
  Merge : Merge
  Unit Delay : UnitDelay  SampleTime=-1  HasFrameUpgradeWarning=on
  Out1 : Outport
  wires:
  In1/1 -> Gain/1
  If/1 -> If Action Subsystem/Action
  If/2 -> If Action Subsystem1/Action
  Unit Delay/1 -> If Action Subsystem1/1(In1)
  If Action Subsystem1/1(Out1) -> Merge/2
  If Action Subsystem/1(Out1) -> Merge/1
  Merge/1 -> Out1/1
  Gain/1 -> Data Type Conversion2/1
  Data Type Conversion2/1 -> Unit Delay/1, If Action Subsystem/1(In1), If/1

== system APLRL2D_avoidance_version/Calculate Observation/Subsystem/If Action Subsystem ==
  In2 : Inport
  In3 : Inport  Port=2
  Action Port : ActionPort  ActionPortLabel=if(u1 > 0 & u1<65535)
  Atan2 : Trigonometry  Operator=atan2
  Constant : Constant  Value=639
  Constant1 : Constant  Value=908.6
  Data Type Conversion1 : DataTypeConversion  OutDataTypeStr=double
  Data Type Conversion2 : DataTypeConversion  OutDataTypeStr=double
  Minus : Sum  Inputs=+-
  Mux : Mux  Inputs=2
  Out1 : Outport
  wires:
  In3/1 -> Minus/2
  Constant/1 -> Minus/1
  Minus/1 -> Atan2/1
  Constant1/1 -> Atan2/2  "1.1e-3's inverse"
  In2/1 -> Data Type Conversion1/1
  Data Type Conversion1/1 -> Mux/1
  Atan2/1 -> Data Type Conversion2/1
  Data Type Conversion2/1 -> Mux/2
  Mux/1 -> Out1/1

== system APLRL2D_avoidance_version/Calculate Observation/Subsystem/If Action Subsystem1 ==
  In1 : Inport
  Action Port : ActionPort  ActionPortLabel=else
  Data Type Conversion3 : DataTypeConversion  OutDataTypeStr=double
  Mux : Mux  Inputs=2
  Out1 : Outport
  wires:
  In1/1 -> Data Type Conversion3/1
  Data Type Conversion3/1 -> Mux/1, Mux/2
  Mux/1 -> Out1/1

== system APLRL2D_avoidance_version/Calculate Observation/Subsystem3/If Action Subsystem ==
  In1 : Inport
  In2 : Inport  Port=2
  Action Port : ActionPort  ActionPortLabel=if(u1 > pi)
  Minus : Sum  Inputs=+-
  Out1 : Outport
  wires:
  In1/1 -> Minus/1
  In2/1 -> Minus/2
  Minus/1 -> Out1/1

== system APLRL2D_avoidance_version/Calculate Observation/Subsystem3/If Action Subsystem1 ==
  In1 : Inport
  In2 : Inport  Port=2
  Action Port : ActionPort  ActionPortLabel=elseif(u1 < -pi)
  Plus : Sum
  Out1 : Outport
  wires:
  In2/1 -> Plus/2
  In1/1 -> Plus/1
  Plus/1 -> Out1/1

== system APLRL2D_avoidance_version/Calculate Observation/Subsystem3/If Action Subsystem2 ==
  In1 : Inport
  Action Port : ActionPort  ActionPortLabel=else
  Out1 : Outport
  wires:
  In1/1 -> Out1/1

== system APLRL2D_avoidance_version/Calculate Reward/If Action Subsystem2/Subsystem4 ==
  In1 : Inport
  Data Type Conversion2 : DataTypeConversion  OutDataTypeStr=uint16
  Gain : Gain  Gain=10
  If : If
  If Action Subsystem : Subsystem  TreatAsAtomicUnit=on
  If Action Subsystem1 : Subsystem  TreatAsAtomicUnit=on
  Merge : Merge
  Unit Delay : UnitDelay  SampleTime=-1  HasFrameUpgradeWarning=on
  Out1 : Outport
  wires:
  In1/1 -> Gain/1
  If/1 -> If Action Subsystem/Action
  If/2 -> If Action Subsystem1/Action
  Unit Delay/1 -> If Action Subsystem1/1(In1)
  If Action Subsystem1/1(Out1) -> Merge/2
  If Action Subsystem/1(Out1) -> Merge/1
  Merge/1 -> Out1/1
  Gain/1 -> Data Type Conversion2/1
  Data Type Conversion2/1 -> Unit Delay/1, If Action Subsystem/1(In1), If/1

== system APLRL2D_avoidance_version/Calculate Reward/Subsystem/If Action Subsystem ==
  In1 : Inport
  Action Port : ActionPort  ActionPortLabel=if(u1 < 0.5)
  Data Type Conversion1 : DataTypeConversion  OutDataTypeStr=double
  Out1 : Outport
  wires:
  In1/1 -> Data Type Conversion1/1
  Data Type Conversion1/1 -> Out1/1

== system APLRL2D_avoidance_version/Calculate Reward/Subsystem/If Action Subsystem1 ==
  In1 : Inport
  Action Port : ActionPort  ActionPortLabel=if(u1 < -1)
  Out1 : Outport
  wires:
  In1/1 -> Out1/1

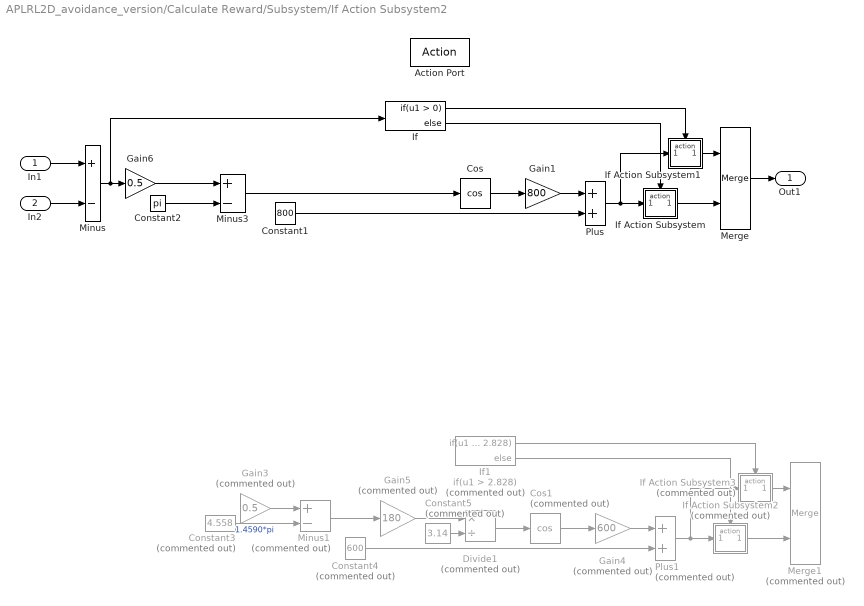
== system APLRL2D_avoidance_version/Calculate Reward/Subsystem/If Action Subsystem2 ==
  In1 : Inport
  In2 : Inport  Port=2
  Action Port : ActionPort  ActionPortLabel=else
  Constant1 : Constant  Value=800
  Constant2 : Constant  Value=pi
  Constant3 : Constant  Commented=on  Value=4.558
  Constant4 : Constant  Commented=on  Value=600
  Constant5 : Constant  Commented=on  Value=3.14
  Cos : Trigonometry  Operator=cos
  Cos1 : Trigonometry  Commented=on  Operator=cos
  Divide1 : Product  Commented=on  Inputs=*/
  Gain1 : Gain  Gain=800
  Gain3 : Gain  Commented=on  Gain=0.5
  Gain4 : Gain  Commented=on  Gain=600
  Gain5 : Gain  Commented=on  Gain=180
  Gain6 : Gain  Gain=0.5
  If : If
  If Action Subsystem : Subsystem  TreatAsAtomicUnit=on
  If Action Subsystem1 : Subsystem  TreatAsAtomicUnit=on
  If Action Subsystem2 : Subsystem  Commented=on  TreatAsAtomicUnit=on
  If Action Subsystem3 : Subsystem  Commented=on  TreatAsAtomicUnit=on
  If1 : If  Commented=on  IfExpression=u1 > 2.828
  Merge : Merge
  Merge1 : Merge  Commented=on
  Minus : Sum  Inputs=+-
  Minus1 : Sum  Commented=on  Inputs=+-
  Minus3 : Sum  Inputs=+-
  Plus : Sum
  Plus1 : Sum  Commented=on
  Out1 : Outport
  wires:
  Minus/1 -> If/1, Gain6/1
  Cos/1 -> Gain1/1
  Constant1/1 -> Plus/2
  Gain1/1 -> Plus/1
  If Action Subsystem1/1(Out1) -> Merge/1
  Plus/1 -> If Action Subsystem1/1(In1), If Action Subsystem/1(In1)
  If Action Subsystem/1(Out1) -> Merge/2
  Merge/1 -> Out1/1
  If1/2 -> If Action Subsystem2/Action
  If Action Subsystem2/1(Out1) -> Merge1/2
  If1/1 -> If Action Subsystem3/Action
  Constant3/1 -> Minus1/2  "1.4590*pi"
  Constant4/1 -> Plus1/2
  Divide1/1 -> Cos1/1
  Constant5/1 -> Divide1/2
  Gain5/1 -> Divide1/1
  If Action Subsystem3/1(Out1) -> Merge1/1
  Cos1/1 -> Gain4/1
  Minus1/1 -> Gain5/1
  Gain4/1 -> Plus1/1
  Gain3/1 -> Minus1/1
  Plus1/1 -> If Action Subsystem3/1(In1), If Action Subsystem2/1(In1)
  In2/1 -> Minus/2
  Constant2/1 -> Minus3/2
  In1/1 -> Minus/1
  Gain6/1 -> Minus3/1
  Minus3/1 -> Cos/1
  If/1 -> If Action Subsystem1/Action
  If/2 -> If Action Subsystem/Action

== system APLRL2D_avoidance_version/Calculate Reward/Subsystem/If Action Subsystem3 ==
  In1 : Inport
  Action Port : ActionPort  ActionPortLabel=else
  If : If
  If Action Subsystem : Subsystem  TreatAsAtomicUnit=on
  If Action Subsystem1 : Subsystem  TreatAsAtomicUnit=on
  Merge : Merge
  Subsystem : Subsystem
  Out1 : Outport
  wires:
  In1/1 -> If/1, Subsystem/1(In1)
  If/1 -> If Action Subsystem/Action
  If/2 -> If Action Subsystem1/Action
  If Action Subsystem/1(Out1) -> Merge/1
  If Action Subsystem1/1(Out1) -> Merge/2
  Merge/1 -> Out1/1
  Subsystem/1(Out1) -> If Action Subsystem1/1(In1), If Action Subsystem/1(In1)

== system APLRL2D_avoidance_version/Calculate Reward/Subsystem/If Action Subsystem4 ==
  In1 : Inport
  Action Port : ActionPort  ActionPortLabel=if(u1 > 1e4)
  Out1 : Outport
  wires:
  In1/1 -> Out1/1

== system APLRL2D_avoidance_version/Calculate Reward/Subsystem/If Action Subsystem5 ==
  In1 : Inport
  Action Port : ActionPort  ActionPortLabel=else
  Out1 : Outport
  wires:
  In1/1 -> Out1/1

== system APLRL2D_avoidance_version/Calculate Reward/Subsystem4/If Action Subsystem ==
  In2 : Inport
  Action Port : ActionPort  ActionPortLabel=if(u1 > 0 & u1<10000)
  Constant : Constant  Value=1000
  Constant1 : Constant
  Data Type Conversion1 : DataTypeConversion  OutDataTypeStr=double
  Data Type Conversion2 : DataTypeConversion  OutDataTypeStr=uint16
  Divide : Product  Inputs=*/
  Gain : Gain  Gain=0.01
  Gain1 : Gain  Gain=1e-4
  Plus : Sum
  Square : Math  Operator=square  SaturateOnIntegerOverflow=on
  Out1 : Outport
  wires:
  In2/1 -> Gain/1
  Data Type Conversion1/1 -> Out1/1
  Gain/1 -> Data Type Conversion2/1
  Square/1 -> Gain1/1
  Constant/1 -> Divide/1
  Divide/1 -> Data Type Conversion1/1
  Data Type Conversion2/1 -> Square/1
  Gain1/1 -> Plus/1
  Constant1/1 -> Plus/2
  Plus/1 -> Divide/2

== system APLRL2D_avoidance_version/Calculate Reward/Subsystem4/If Action Subsystem1 ==
  In1 : Inport
  Action Port : ActionPort  ActionPortLabel=else
  Data Type Conversion3 : DataTypeConversion  OutDataTypeStr=double
  Out1 : Outport
  wires:
  In1/1 -> Data Type Conversion3/1
  Data Type Conversion3/1 -> Out1/1

== system APLRL2D_avoidance_version/Calculate Reward/Subsystem4/If Action Subsystem2 ==
  In1 : Inport
  Action Port : ActionPort  ActionPortLabel=if(u1 > 0 & u1<3000)
  Data Type Conversion3 : DataTypeConversion  OutDataTypeStr=double
  Out1 : Outport
  wires:
  In1/1 -> Data Type Conversion3/1
  Data Type Conversion3/1 -> Out1/1

== system APLRL2D_avoidance_version/Calculate Reward/Subsystem4/If Action Subsystem3 ==
  In1 : Inport
  Action Port : ActionPort  ActionPortLabel=else
  Data Type Conversion3 : DataTypeConversion  OutDataTypeStr=double
  Out1 : Outport
  wires:
  In1/1 -> Data Type Conversion3/1
  Data Type Conversion3/1 -> Out1/1
